simulink model "rtwdemo_capi_bot"  (Simulink 7.6)
settings: Solver=FixedStepDiscrete  StartTime=0.0  StopTime=10.0  RelTol=1e-3  SampleTimeConstraint=STIndependent
PostLoadFcn:
  | rtwdemo_capi_data
values from neighbouring files (symbols this model uses):
  Ki = Simulink.Parameter    [rtwdemo_capi_data.m]
  Kp = Simulink.Parameter    [rtwdemo_capi_data.m]
Description:
  | Target-Based Data Interface: C-API Data Definition File (Model Reference Component)
settings Model: Creator=The MathWorks Inc.  ExtModeTrigMode=oneshot  ExtModeArmWhenConnect=off  ExtModeAutoUpdateStatusClock=off
settings DataIOCC: LimitDataPoints=off  SaveFormat=Structure  SaveOutput=off  SaveTime=off  SignalLoggingName=sigsOut
settings OptimizationCC: InlineParams=on  InlineInvariantSignals=on  StateBitsets=on  DataBitsets=on  UseTempVars=on  EfficientFloat2IntCast=on
settings DebuggingCC: CheckExecutionContextPreStartOutputMsg=on  CheckExecutionContextRuntimeOutputMsg=on  SolverPrmCheckMsg=none  UnconnectedInputMsg=none  UnconnectedOutputMsg=none  UnconnectedLineMsg=none  ModelReferenceSymbolNameMessage=none  StrictBusMsg=ErrorOnBusTreatedAsVector
settings HardwareCC: ProdIntDivRoundTo=Zero  ProdEndianess=LittleEndian  ProdHWDeviceType=Generic->32-bit Embedded Processor  TargetHWDeviceType=Generic->32-bit Embedded Processor
settings ModelReferenceCC: ModelReferencePassRootInputsByReference=off
settings RTWCC: TLCOptions=-p0 -aWarnNonSaturatedBlocks=0  GenerateReport=on  RTWVerbose=off  ProcessScript=grt_make_rtw_hook  LaunchReport=on
settings CodeAppCC: ForceParamTrailComments=on
settings GRTTargetCC: RTWCAPISignals=on  RTWCAPIParams=on  RTWCAPIStates=on

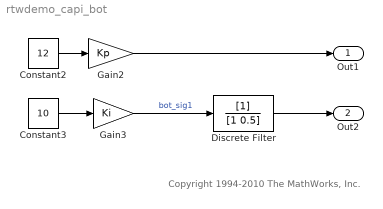
== system rtwdemo_capi_bot ==
  note: Copyright 1994-2010 The MathWorks, Inc.
  Constant2 : Constant  Value=12
  Constant3 : Constant  Value=10
  Discrete Filter : DiscreteFilter  StateIdentifier=bot_state
  Gain2 : Gain  Gain=Kp  SaturateOnIntegerOverflow=on  OutDataTypeStr=Inherit: Same as input  ParamDataTypeStr=Inherit: Same as input
  Gain3 : Gain  Gain=Ki  SaturateOnIntegerOverflow=on  OutDataTypeStr=Inherit: Same as input  ParamDataTypeStr=Inherit: Same as input
  Out1 : Outport
  Out2 : Outport  Port=2
  wires:
  Constant2/1 -> Gain2/1
  Gain2/1 -> Out1/1
  Constant3/1 -> Gain3/1
  Gain3/1 -> Discrete Filter/1  "bot_sig1"
  Discrete Filter/1 -> Out2/1
